simulink model "VTVPB2"  (Simulink 8.5)
settings: Solver=ode3  StartTime=0.0  StopTime=10.0  FixedStep=0.1  RelTol=1e-3
settings Model: Creator=ASUS  LastModifiedBy=ASUS
settings DataIOCC: SignalLoggingSaveFormat=Dataset
settings OptimizationCC: ExpressionDepthLimit=128
settings DebuggingCC: UnderspecifiedInitializationDetection=Simplified  MergeDetectMultiDrivingBlocksExec=error  FcnCallInpInsideContextMsg=EnableAllAsError  StateNameClashWarn=none
settings GRTTargetCC: CombineOutputUpdateFcns=on  GRTInterface=off

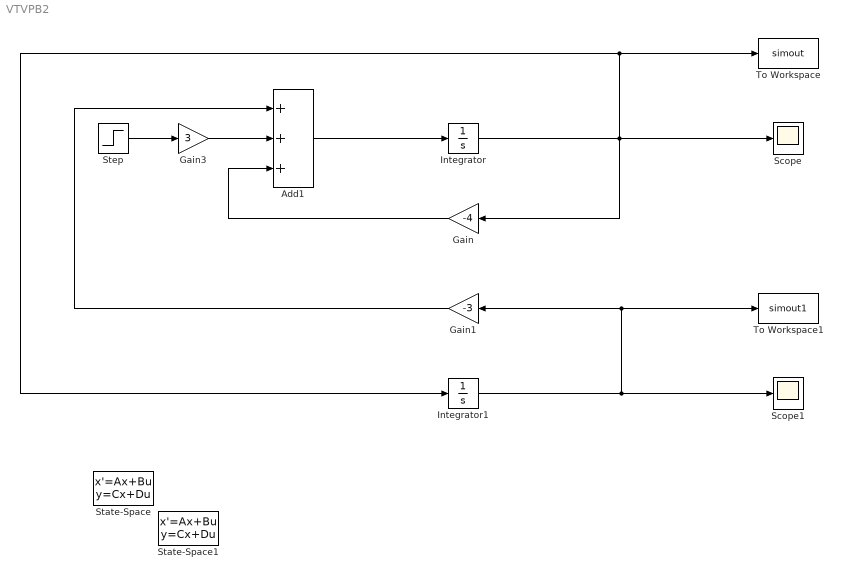
== system VTVPB2 ==
  Add1 : Sum  Inputs=+++
  Gain : Gain  Gain=-4
  Gain1 : Gain  Gain=-3
  Gain3 : Gain  Gain=3
  Integrator : Integrator
  Integrator1 : Integrator  InitialCondition=0.5
  Scope : Scope
  Scope1 : Scope
  State-Space : StateSpace  X0=0
  State-Space1 : StateSpace  X0=0
  Step : Step  SampleTime=0
  To Workspace : ToWorkspace  VariableName=simout  SampleTime=-1
  To Workspace1 : ToWorkspace  VariableName=simout1  SampleTime=-1
  wires:
  Integrator/1 -> Gain/1, Scope/1, To Workspace/1, Integrator1/1
  Add1/1 -> Integrator/1
  Step/1 -> Gain3/1
  Integrator1/1 -> Gain1/1, To Workspace1/1, Scope1/1
  Gain3/1 -> Add1/2
  Gain/1 -> Add1/3
  Gain1/1 -> Add1/1
